simulink model "sldemo_tonegen"  (Simulink 7.6)
settings: Solver=FixedStepDiscrete  SolverMode=SingleTasking  StartTime=0  StopTime=30  FixedStep=1/256  RelTol=1e-3
StartFcn:
  | if exist('tonegen_ploth')
  |   if ishghandle(tonegen_ploth,'figure'), close(tonegen_ploth); end
  |   clear tonegen_ploth
  | end
StopFcn:
  | if exist('tonegenOut')
  |   tonegen_ploth = figure;
  |   subplot(3,1,1), plot(tonegenOut.time, tonegenOut.signals(1).values); grid
  |   title('Difference between direct look-up and reference signal');
  |   subplot(3,1,2), plot(tonegenOut.time, tonegenOut.signals(2).values); grid
  |   title('Difference between interpolated look-up and reference signal');
  |   subplot(3,1,3), plot(tonegenOut.time, tonegenOut.signals(3).values); grid
  |   title('Difference between CORDIC sine and reference signal');
  | end
libraries: simulink x1
Description:
  | Tone Generation Algorithm Comparison
  | 
  | Uses a sampled sine wave designed using ssinthd.m to see how it works as a
  | direct lookup, with linear interpolation and with CORDIC approximation. This
  | model compares the output of the floating point tables to the sin() function.
  | As expected from the THD calculations, the linear interpolation has a lower
  | error than the direct table lookup in comparison to the sin() function. The
  | CORDIC approximation has a lower error than linear interpolation.
CloseFcn:
  | if exist('tonegen_ploth')
  |   if ishghandle(tonegen_ploth,'figure'), close(tonegen_ploth); end
  |   clear tonegen_ploth
  |   if exist('tonegenOut'), clear tonegenOut; end
  | end
settings Model: Creator=The MathWorks Inc.  ExtModeAutoUpdateStatusClock=off
settings DataIOCC: LimitDataPoints=off  SaveFormat=StructureWithTime  SaveTime=off  OutputSaveName=tonegenOut  SignalLoggingName=sigsOut
settings OptimizationCC: InlineInvariantSignals=on  InitFltsAndDblsToZero=on  BufferReusableBoundary=off
settings DebuggingCC: SaveWithParameterizedLinksMsg=none  CheckExecutionContextPreStartOutputMsg=on  CheckExecutionContextRuntimeOutputMsg=on  SignalResolutionControl=TryResolveAllWithWarning  SolverPrmCheckMsg=none  MultiTaskDSMMsg=warning  MultiTaskCondExecSysMsg=none  BusObjectLabelMismatch=none
settings HardwareCC: TargetUnknown=on
settings RTWCC: IncludeERTFirstTime=on
settings CodeAppCC: CustomSymbolStrFcn=$F$N$M
settings GRTTargetCC: TargetFcnLib=ansi_tfl_tmw.mat

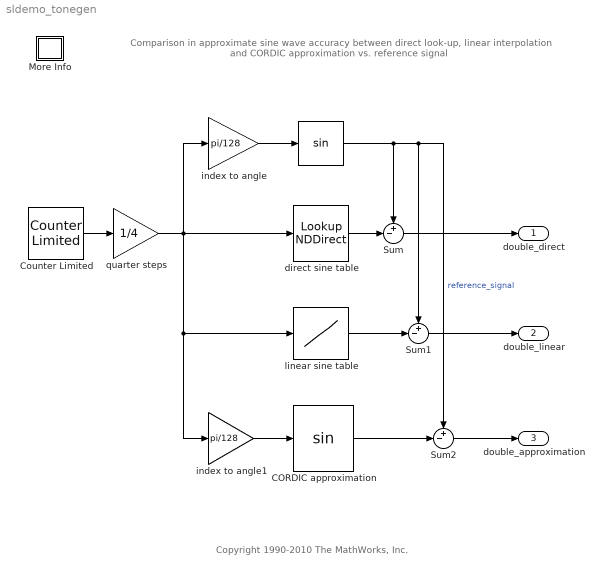
== system sldemo_tonegen ==
  note: Comparison in approximate sine wave accuracy between
      | direct look-up, linear interpolation and CORDIC approximation
      |  vs. reference signal
  note: Copyright 1990-2010 The MathWorks, Inc.
  " " : Trigonometry  NumberOfIterations=50
  CORDIC approximation : Trigonometry  ApproximationMethod=CORDIC  NumberOfIterations=50
  Counter Limited : simulink/Sources/Counter Limited  SystemSampleTime=-1  uplimit=1023  tsamp=-1
  More Info : Subsystem
      settings: OpenFcn=showdemo('sldemo_wavethd_script')
      mask Display: disp('?')
  Sum : Sum  Inputs=+-|
  Sum1 : Sum  Inputs=+-|
  Sum2 : Sum  Inputs=+-|
  direct sine table : LookupNDDirect  NumberOfTableDimensions=1  Table=sin( 2*pi * (0:255)/256)'
  index to angle : Gain  Gain=pi/128  OutDataTypeStr=double
  index to angle1 : Gain  Gain=pi/128  OutDataTypeStr=double
  linear sine table : Lookup_n-D  NumberOfTableDimensions=1  BreakpointsForDimension1=[0:256]  IndexSearchMethod=Linear search  BeginIndexSearchUsingPreviousIndexResult=on  Table=sin( 2*pi * (0:256)/256 )'  ExtrapMethod=None - Clip  ActionForOutOfRangeInput=Warning  InputSameDT=on
  quarter steps : Gain  Gain=1/4  OutDataTypeStr=float('double')
  double_direct : Outport
  double_linear : Outport  Port=2
  double_approximation : Outport  Port=3
  wires:
  Counter Limited/1 -> quarter steps/1
  quarter steps/1 -> direct sine table/1, linear sine table/1, index to angle1/1, index to angle/1
  " "/1 -> Sum/1, Sum1/1, Sum2/1  "reference_signal"
  direct sine table/1 -> Sum/2
  linear sine table/1 -> Sum1/2
  Sum/1 -> double_direct/1
  Sum1/1 -> double_linear/1
  CORDIC approximation/1 -> Sum2/2
  Sum2/1 -> double_approximation/1
  index to angle1/1 -> CORDIC approximation/1
  index to angle/1 -> " "/1

== system sldemo_tonegen/More Info ==
